simulink model "wave_simulate"  (R2014b)
settings: Solver=ode45  StartTime=0.0  StopTime=10.0  RelTol=1e-3
libraries: xbsIndex_r4 x1, simulink_extras x1
settings Model: Creator=mtech  LastModifiedBy=mtech

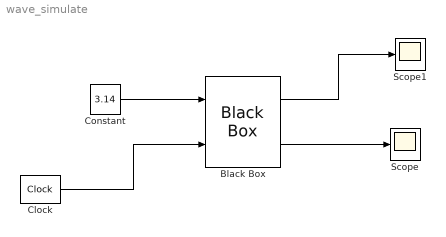
== system wave_simulate ==
  Black Box : xbsIndex_r4/Black Box  init_code=sin_cos_module_config  sim_method=ISE Simulator  verbose=off  block_type=blackbox2
  Clock : simulink_extras/Flip Flops/Clock  period=2
  Constant : Constant  Value=3.14  SampleTime=1
  Scope : Scope
  Scope1 : Scope
  wires:
  Constant/1 -> Black Box/1
  Clock/1 -> Black Box/2
  Black Box/2 -> Scope/1
  Black Box/1 -> Scope1/1
